simulink subsystem "rss_PwrTubPCBTempHiLvl1Dia"  (R2023a)
settings: Solver=VariableStepAuto  StartTime=0.0  StopTime=10.0  RelTol=1e-3
undefined symbols (not defined in the file): ENM_TYPE_FALT, Gu16_ctPCBTempHiLvl1ConfCnt_C, Gu16_ctPCBTempHiLvl1RcvyCnt_C, Gu16_ctPwrTubTempHiLvl1ConfCnt_C, Gu16_ctPwrTubTempHiLvl1RcvyCnt_C, Gu8_tPCBTempHiLvl1ConfTrs_C, Gu8_tPCBTempHiLvl1RcvyTrs_C, Gu8_tPwrTubTempHiLvl1ConfTrs_C, Gu8_tPwrTubTempHiLvl1RcvyTrs_C
libraries: vhit_control_library x2, lib_fault_definiteness x1
settings Model: Creator=xiaoqiang.yuan  LastModifiedBy=xiaoqiang.yuan

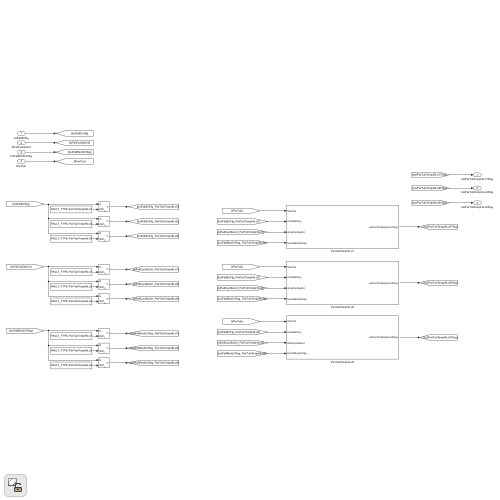
[thumbnail: Simulink's stored preview of the top-level diagram]
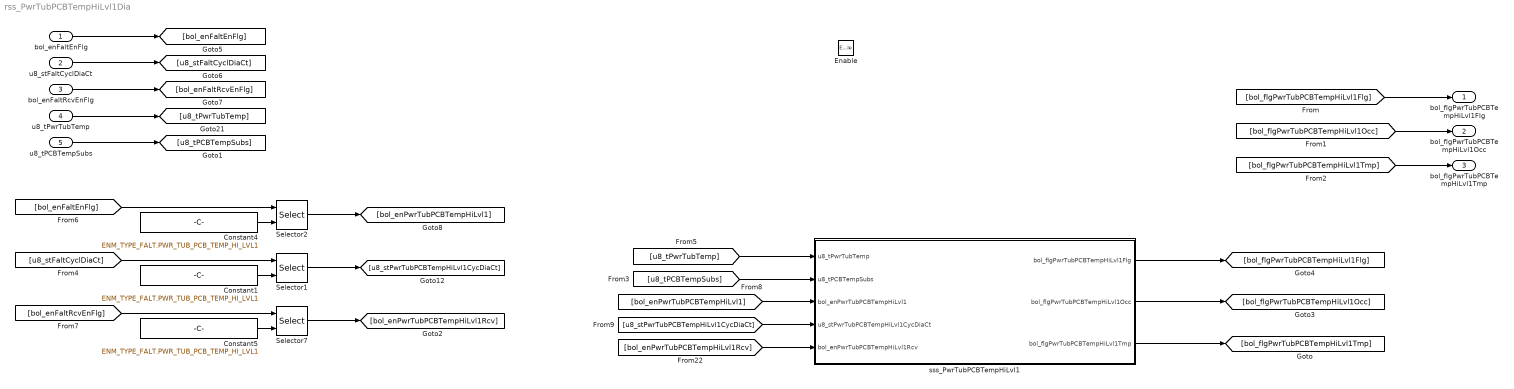
== system rss_PwrTubPCBTempHiLvl1Dia ==
  bol_enFaltEnFlg : Inport  OutDataTypeStr=boolean
  u8_stFaltCyclDiaCt : Inport  Port=2  OutDataTypeStr=uint8
  bol_enFaltRcvEnFlg : Inport  Port=3  OutDataTypeStr=boolean
  u8_tPwrTubTemp : Inport  Port=4  OutDataTypeStr=dt_Temp_u8p0bn40
  u8_tPCBTempSubs : Inport  Port=5  OutDataTypeStr=dt_Temp_u8p0bn40
  Enable : EnablePort
  Constant1 : Constant  Value=ENM_TYPE_FALT.PWR_TUB_PCB_TEMP_HI_LVL1
  Constant4 : Constant  Value=ENM_TYPE_FALT.PWR_TUB_PCB_TEMP_HI_LVL1
  Constant5 : Constant  Value=ENM_TYPE_FALT.PWR_TUB_PCB_TEMP_HI_LVL1
  Selector1 : Selector  IndexMode=Zero-based  InputPortWidth=Cdbl_numFaltDiaNum  IndexOptions=Index vector (port)  Indices=[1 3]  OutputSizes=1
  Selector2 : Selector  IndexMode=Zero-based  InputPortWidth=Cdbl_numFaltDiaNum  IndexOptions=Index vector (port)  Indices=[1 3]  OutputSizes=1
  Selector7 : Selector  IndexMode=Zero-based  InputPortWidth=Cdbl_numFaltDiaNum  IndexOptions=Index vector (port)  Indices=[1 3]  OutputSizes=1
  sss_PwrTubPCBTempHiLvl1 : Subsystem
  bol_flgPwrTubPCBTempHiLvl1Flg : Outport  OutDataTypeStr=boolean
  bol_flgPwrTubPCBTempHiLvl1Occ : Outport  Port=2  OutDataTypeStr=boolean
  bol_flgPwrTubPCBTempHiLvl1Tmp : Outport  Port=3  OutDataTypeStr=boolean
  wires:
  [bol_flgPwrTubPCBTempHiLvl1Flg] -> bol_flgPwrTubPCBTempHiLvl1Flg/1
  u8_tPwrTubTemp/1 -> [u8_tPwrTubTemp]
  Selector2/1 -> [bol_enPwrTubPCBTempHiLvl1]
  [bol_enFaltEnFlg] -> Selector2/1
  [bol_enPwrTubPCBTempHiLvl1] -> sss_PwrTubPCBTempHiLvl1/3(bol_enPwrTubPCBTempHiLvl1)
  Constant4/1 -> Selector2/2
  [u8_stPwrTubPCBTempHiLvl1CycDiaCt] -> sss_PwrTubPCBTempHiLvl1/4(u8_stPwrTubPCBTempHiLvl1CycDiaCt)
  [u8_tPwrTubTemp] -> sss_PwrTubPCBTempHiLvl1/1(u8_tPwrTubTemp)
  bol_enFaltEnFlg/1 -> [bol_enFaltEnFlg]
  bol_enFaltRcvEnFlg/1 -> [bol_enFaltRcvEnFlg]
  u8_stFaltCyclDiaCt/1 -> [u8_stFaltCyclDiaCt]
  [bol_enPwrTubPCBTempHiLvl1Rcv] -> sss_PwrTubPCBTempHiLvl1/5(bol_enPwrTubPCBTempHiLvl1Rcv)
  Selector1/1 -> [u8_stPwrTubPCBTempHiLvl1CycDiaCt]
  Constant1/1 -> Selector1/2
  [u8_stFaltCyclDiaCt] -> Selector1/1
  Selector7/1 -> [bol_enPwrTubPCBTempHiLvl1Rcv]
  Constant5/1 -> Selector7/2
  [bol_enFaltRcvEnFlg] -> Selector7/1
  sss_PwrTubPCBTempHiLvl1/1(bol_flgPwrTubPCBTempHiLvl1Flg) -> [bol_flgPwrTubPCBTempHiLvl1Flg]
  u8_tPCBTempSubs/1 -> [u8_tPCBTempSubs]
  [u8_tPCBTempSubs] -> sss_PwrTubPCBTempHiLvl1/2(u8_tPCBTempSubs)
  sss_PwrTubPCBTempHiLvl1/2(bol_flgPwrTubPCBTempHiLvl1Occ) -> [bol_flgPwrTubPCBTempHiLvl1Occ]
  [bol_flgPwrTubPCBTempHiLvl1Occ] -> bol_flgPwrTubPCBTempHiLvl1Occ/1
  [bol_flgPwrTubPCBTempHiLvl1Tmp] -> bol_flgPwrTubPCBTempHiLvl1Tmp/1
  sss_PwrTubPCBTempHiLvl1/3(bol_flgPwrTubPCBTempHiLvl1Tmp) -> [bol_flgPwrTubPCBTempHiLvl1Tmp]

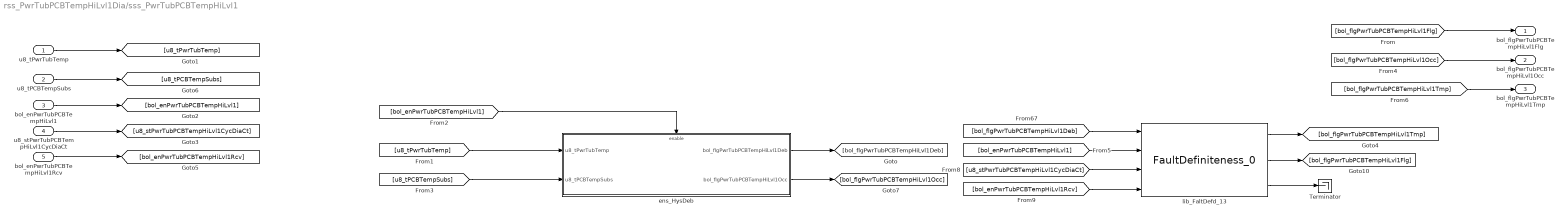
== system rss_PwrTubPCBTempHiLvl1Dia/sss_PwrTubPCBTempHiLvl1 ==
  u8_tPwrTubTemp : Inport
  u8_tPCBTempSubs : Inport  Port=2
  bol_enPwrTubPCBTempHiLvl1 : Inport  Port=3
  u8_stPwrTubPCBTempHiLvl1CycDiaCt : Inport  Port=4
  bol_enPwrTubPCBTempHiLvl1Rcv : Inport  Port=5
  Terminator : Terminator
  ens_HysDeb : Subsystem
  lib_FaltDefd_13 : lib_fault_definiteness/FaultDefiniteness_0  lb_FaltWaitRecvCnt=Gu16_ctPwrTubTempHiLvl1ConfCnt_C
  bol_flgPwrTubPCBTempHiLvl1Flg : Outport
  bol_flgPwrTubPCBTempHiLvl1Occ : Outport  Port=2
  bol_flgPwrTubPCBTempHiLvl1Tmp : Outport  Port=3
  wires:
  [bol_flgPwrTubPCBTempHiLvl1Tmp] -> bol_flgPwrTubPCBTempHiLvl1Tmp/1
  [bol_flgPwrTubPCBTempHiLvl1Occ] -> bol_flgPwrTubPCBTempHiLvl1Occ/1
  ens_HysDeb/2(bol_flgPwrTubPCBTempHiLvl1Occ) -> [bol_flgPwrTubPCBTempHiLvl1Occ]
  [u8_tPCBTempSubs] -> ens_HysDeb/2(u8_tPCBTempSubs)
  u8_tPCBTempSubs/1 -> [u8_tPCBTempSubs]
  lib_FaltDefd_13/1 -> [bol_flgPwrTubPCBTempHiLvl1Tmp]
  lib_FaltDefd_13/2 -> [bol_flgPwrTubPCBTempHiLvl1Flg]
  lib_FaltDefd_13/3 -> Terminator/1
  [bol_enPwrTubPCBTempHiLvl1] -> ens_HysDeb/Enable
  [u8_tPwrTubTemp] -> ens_HysDeb/1(u8_tPwrTubTemp)
  ens_HysDeb/1(bol_flgPwrTubPCBTempHiLvl1Deb) -> [bol_flgPwrTubPCBTempHiLvl1Deb]
  bol_enPwrTubPCBTempHiLvl1Rcv/1 -> [bol_enPwrTubPCBTempHiLvl1Rcv]
  u8_stPwrTubPCBTempHiLvl1CycDiaCt/1 -> [u8_stPwrTubPCBTempHiLvl1CycDiaCt]
  bol_enPwrTubPCBTempHiLvl1/1 -> [bol_enPwrTubPCBTempHiLvl1]
  [bol_flgPwrTubPCBTempHiLvl1Flg] -> bol_flgPwrTubPCBTempHiLvl1Flg/1
  u8_tPwrTubTemp/1 -> [u8_tPwrTubTemp]
  [bol_enPwrTubPCBTempHiLvl1Rcv] -> lib_FaltDefd_13/4
  [u8_stPwrTubPCBTempHiLvl1CycDiaCt] -> lib_FaltDefd_13/3
  [bol_enPwrTubPCBTempHiLvl1] -> lib_FaltDefd_13/2
  [bol_flgPwrTubPCBTempHiLvl1Deb] -> lib_FaltDefd_13/1

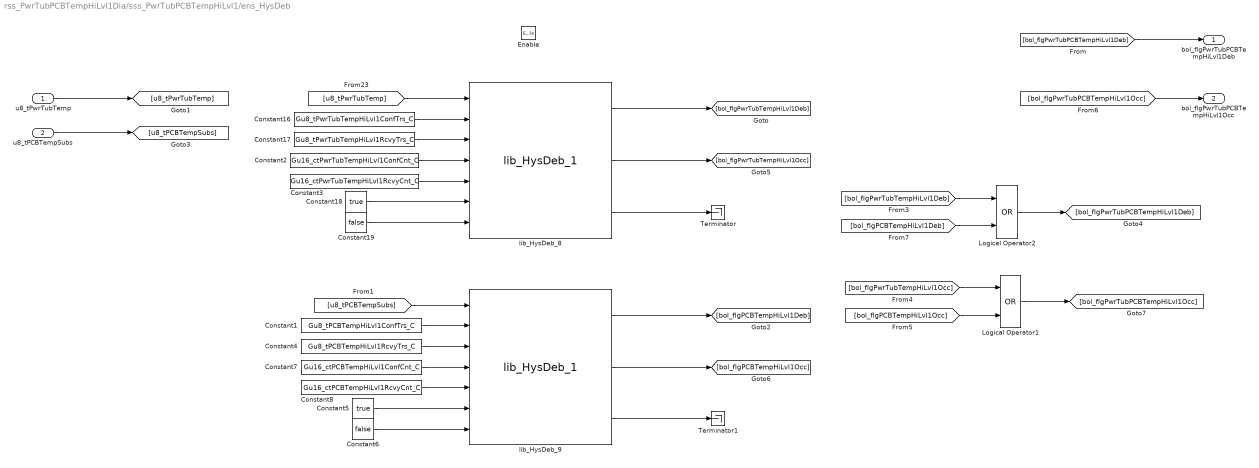
== system rss_PwrTubPCBTempHiLvl1Dia/sss_PwrTubPCBTempHiLvl1/ens_HysDeb ==
  u8_tPwrTubTemp : Inport
  u8_tPCBTempSubs : Inport  Port=2
  Enable : EnablePort
  Constant1 : Constant  Value=Gu8_tPCBTempHiLvl1ConfTrs_C
  Constant16 : Constant  Value=Gu8_tPwrTubTempHiLvl1ConfTrs_C
  Constant17 : Constant  Value=Gu8_tPwrTubTempHiLvl1RcvyTrs_C
  Constant18 : Constant  Value=true  OutDataTypeStr=boolean
  Constant19 : Constant  Value=false  OutDataTypeStr=boolean
  Constant2 : Constant  Value=Gu16_ctPwrTubTempHiLvl1ConfCnt_C
  Constant3 : Constant  Value=Gu16_ctPwrTubTempHiLvl1RcvyCnt_C
  Constant4 : Constant  Value=Gu8_tPCBTempHiLvl1RcvyTrs_C
  Constant5 : Constant  Value=true  OutDataTypeStr=boolean
  Constant6 : Constant  Value=false  OutDataTypeStr=boolean
  Constant7 : Constant  Value=Gu16_ctPCBTempHiLvl1ConfCnt_C
  Constant8 : Constant  Value=Gu16_ctPCBTempHiLvl1RcvyCnt_C
  Logical Operator1 : Logic  Operator=OR  AllPortsSameDT=off  OutDataTypeStr=boolean
  Logical Operator2 : Logic  Operator=OR  AllPortsSameDT=off  OutDataTypeStr=boolean
  Terminator : Terminator
  Terminator1 : Terminator
  lib_HysDeb_8 : vhit_control_library/lib_HysDeb_1  lb_parInitOutp=0
  lib_HysDeb_9 : vhit_control_library/lib_HysDeb_1  lb_parInitOutp=0
  bol_flgPwrTubPCBTempHiLvl1Deb : Outport
  bol_flgPwrTubPCBTempHiLvl1Occ : Outport  Port=2
  wires:
  [bol_flgPCBTempHiLvl1Deb] -> Logical Operator2/2
  [bol_flgPwrTubTempHiLvl1Deb] -> Logical Operator2/1
  Logical Operator2/1 -> [bol_flgPwrTubPCBTempHiLvl1Deb]
  [bol_flgPwrTubPCBTempHiLvl1Occ] -> bol_flgPwrTubPCBTempHiLvl1Occ/1
  Logical Operator1/1 -> [bol_flgPwrTubPCBTempHiLvl1Occ]
  [bol_flgPCBTempHiLvl1Occ] -> Logical Operator1/2
  [bol_flgPwrTubTempHiLvl1Occ] -> Logical Operator1/1
  lib_HysDeb_9/2 -> [bol_flgPCBTempHiLvl1Occ]
  lib_HysDeb_9/3 -> Terminator1/1
  lib_HysDeb_8/2 -> [bol_flgPwrTubTempHiLvl1Occ]
  lib_HysDeb_8/1 -> [bol_flgPwrTubTempHiLvl1Deb]
  lib_HysDeb_8/3 -> Terminator/1
  [u8_tPCBTempSubs] -> lib_HysDeb_9/1
  Constant7/1 -> lib_HysDeb_9/4
  Constant1/1 -> lib_HysDeb_9/2
  lib_HysDeb_9/1 -> [bol_flgPCBTempHiLvl1Deb]
  u8_tPCBTempSubs/1 -> [u8_tPCBTempSubs]
  Constant5/1 -> lib_HysDeb_9/6
  Constant6/1 -> lib_HysDeb_9/7
  Constant4/1 -> lib_HysDeb_9/3
  Constant8/1 -> lib_HysDeb_9/5
  Constant3/1 -> lib_HysDeb_8/5
  Constant2/1 -> lib_HysDeb_8/4
  Constant19/1 -> lib_HysDeb_8/7
  Constant18/1 -> lib_HysDeb_8/6
  Constant17/1 -> lib_HysDeb_8/3
  Constant16/1 -> lib_HysDeb_8/2
  [u8_tPwrTubTemp] -> lib_HysDeb_8/1
  u8_tPwrTubTemp/1 -> [u8_tPwrTubTemp]
  [bol_flgPwrTubPCBTempHiLvl1Deb] -> bol_flgPwrTubPCBTempHiLvl1Deb/1
